simulink model "Linear_State_Space_Model"  (R2021a)
settings: Solver=VariableStepAuto  StartTime=0.0  StopTime=10.0  RelTol=1e-3
values from neighbouring files (symbols this model uses):
  A = [0 0 0 1 0 0;0 0 0 0 1 0;0 0 0 0 0 1;0 0 0 0 0 0;0 0 0 0 0 0;0 0 0 0 0 0]    [Statematrix.m]    (also in parameter.m)
  B = [0 0 0 0;0 0 0 0;0 0 0 0;-kt/jy -kt/jy kt/jy kt/jy;L*kf/jp -L*kf/jp 0 0;0 0 L*kf/jr -L*kf/jr]    [Statematrix.m]    (also in parameter.m)
  C = [1 0 0 0 0 0;0 1 0 0 0 0;0 0 1 0 0 0]    [Statematrix.m]    (also in parameter.m)
  D = [0 0 0 0;0 0 0 0;0 0 0 0]    [Statematrix.m]    (also in parameter.m)
settings Model: Creator=44743  LastModifiedBy=44743

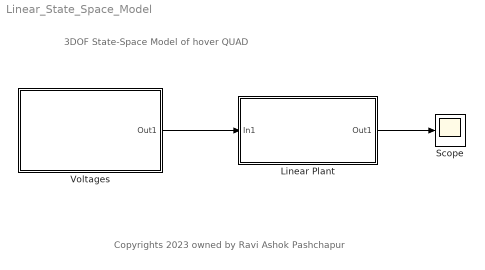
== system Linear_State_Space_Model ==
  note: 3DOF State-Space Model of hover QUAD
  note: Copyrights 2023 owned by Ravi Ashok Pashchapur
  Linear Plant : Subsystem
  Scope : Scope
  Voltages : Subsystem
  wires:
  Linear Plant/1(Out1) -> Scope/1
  Voltages/1(Out1) -> Linear Plant/1(In1)

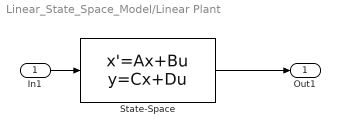
== system Linear_State_Space_Model/Linear Plant ==
  In1 : Inport
  State-Space : StateSpace  A=A  B=B  C=C  D=D  InitialCondition=0
  Out1 : Outport
  wires:
  In1/1 -> State-Space/1
  State-Space/1 -> Out1/1

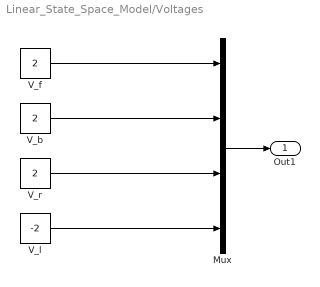
== system Linear_State_Space_Model/Voltages ==
  Mux : Mux
  V_b : Constant  Value=2
  V_f : Constant  Value=2
  V_l : Constant  Value=-2
  V_r : Constant  Value=2
  Out1 : Outport
  wires:
  V_r/1 -> Mux/3
  V_b/1 -> Mux/2
  V_f/1 -> Mux/1
  V_l/1 -> Mux/4
  Mux/1 -> Out1/1
